simulink model "GWOpss"  (R2025a)
settings: Solver=VariableStepAuto  StartTime=0.0  StopTime=30  RelTol=1e-3
undefined symbols (not defined in the file or in its folder): D1, Delta
libraries: spsExcitationSystemLib x1, spsHydraulicTurbineandGovernorLib x1, spsSynchronousMachinepuStandardLib x1, spsThreePhaseParallelRLCLoadLib x1, spsThreePhaseSeriesRLCBranchLib x1, spsThreePhaseTransformerTwoWindingsLib x1, spsThreePhaseFaultLib x1, spsThreePhaseSourceLib x1, sps_lib x1
settings Model: NumberOfSteps=3  Creator=Amal Ibrahim  LastModifiedBy=Amal Ibrahim
settings DataIOCC: ReturnWorkspaceOutputs=off

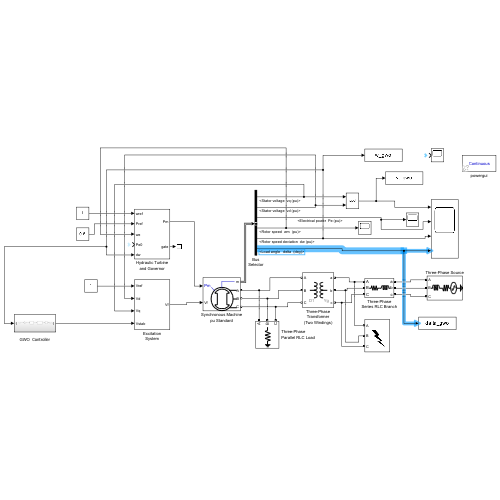
[thumbnail: Simulink's stored preview of the top-level diagram]
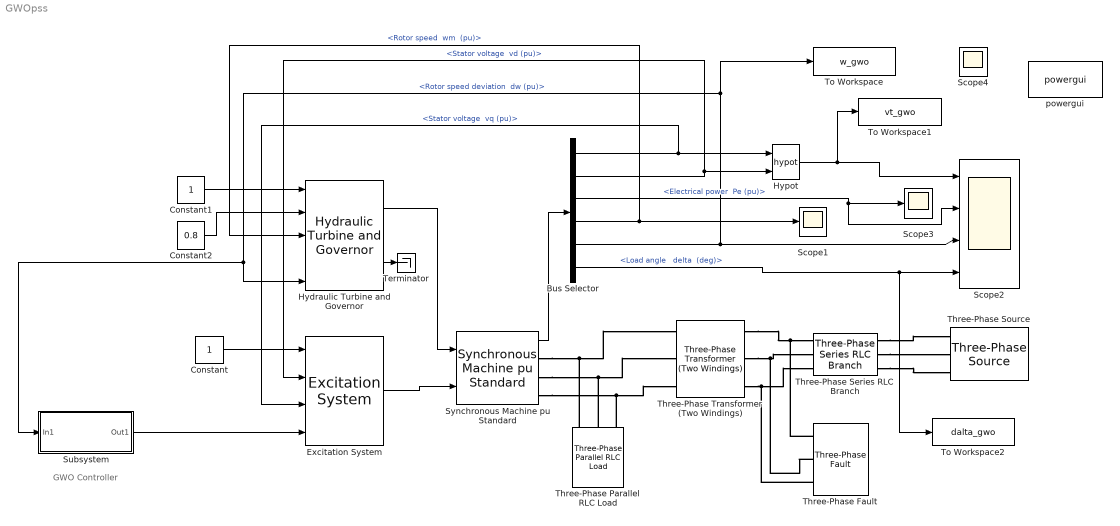
== system GWOpss ==
  note: GWO Controller
  Bus Selector : BusSelector  OutputSignals="dq0 components.Stator voltage  vq (pu),dq0 components.Stator voltage  vd (pu),Mechanical.Electrical power  Pe (pu),Mechanical.Rotor speed  wm  (pu),Mechanical.Rotor speed deviation  dw (pu),Load angle   delta  (deg)"
  Constant : Constant
  Constant1 : Constant
  Constant2 : Constant  Value=0.8
  Excitation System : spsExcitationSystemLib/Excitation System  tr=20e-3  reg=[ 300, 0.001 ]  exc=[ 1, 0 ]  tgr=[ 0, 0 ]  damp=[ 0.01, 0.1 ]  sat=[ 0, 0 ]  lim=[ -11.5, 11.5, 0 ]  v0="[1.0  1.0]"
      settings: LibrarySourceBlock=sps_lib/Electrical Machines/Synchronous Machine Control/Excitation System
  Hydraulic Turbine and Governor : spsHydraulicTurbineandGovernorLib/Hydraulic Turbine and Governor  sm="[ 10/3  0.07 ]"  gate="[  0.01  0.97518  -0.1  0.1 ]"  reg="[  0.05  1.163  0.105  0  0.01  ]"  hyd="[  0  2.67  ]"  dref=0  po=0.8
      settings: LibrarySourceBlock=|
      | sps_lib/Electrical Machines/Synchronous Machine Control/Hydraulic Turbine
      | and Governor
  Hypot : Math  Operator=hypot
  Scope1 : Scope
      settings: ActiveDisplayYMinimum=0.97376212341853119  ActiveDisplayYMaximum=1.0225346527897865
  Scope2 : Scope  NumInputPorts=4
      settings: ActiveDisplayYMinimum=0.13824524933651339  ActiveDisplayYMaximum=1.3474277133856665  DataLoggingVariableName=ScopeData2
  Scope3 : Scope
      settings: ActiveDisplayYMinimum=-1.8399343461680453  ActiveDisplayYMaximum=3.3298477716567159
  Scope4 : Scope
      settings: ActiveDisplayYMinimum=-0.026237876581468769  ActiveDisplayYMaximum=0.022534652789786613  DataLoggingVariableName=ScopeData3
  Subsystem : Subsystem
  Synchronous Machine pu Standard : spsSynchronousMachinepuStandardLib/Synchronous Machine pu Standard  PresetModel=No  MechanicalLoad=Mechanical power Pm  ShowDetailedParameters=on  RotorType=Salient-pole  Units=per unit standard parameters  MeasurementBus=off  NominalParameters=[200E6 13800 60]  Reactances1=[ 1.81, 0.3, 0.23, 1.76, 0.65, 0.25, 0.15 ]  Reactances2=[1.305 0.296 0.252 0.474 0.243 0.18]  dAxisTimeConstants=Short-circuit  qAxisTimeConstants=Open-circuit  TimeConstants1="[ 4.4849  0.0681  0.1  ]"  TimeConstants2=[ 8.0, 0.03, 1.0, 0.07 ]  TimeConstants3="[  4.49  0.0681  0.0513  ]"  TimeConstants4=[ 8.0, 0.03, 0.3371, 0.0295 ]  TimeConstants5=[ 1.01, 0.053, 0.1 ]  TimeConstants6=[ 1.3201, 0.023, 1.0, 0.07 ]  TimeConstants7=[0.012 0.003 0.003]  TimeConstants8=[ 1.3201, 0.0231, 0.3371, 0.0295 ]  StatorResistance=0.037875  Mechanical=[3.2 0 32]  PolePairs=20  InitialConditions="[ 0  0  0  0  0  0  0  0  1 ]"  SetSaturation=off  Saturation=[0.6404,0.7127,0.8441,0.9214,0.9956,1.082,1.19,1.316,1.457;0.7,0.7698,0.8872,0.9466,0.9969,1.046,1.1,1.151,1.201]  LoadFlowParameters=[1,0,0,0,0]  TsPowergui=0  TsBlock=-1  IterativeModel=Trapezoidal non iterative  IterativeDiscreteModel=Trapezoidal non iterative  BusType=PV  Pref=0  Qref=0  Qmin=-inf  Qmax=inf  PLF=0  QLF=0
  Terminator : Terminator
  Three-Phase Parallel RLC Load : spsThreePhaseParallelRLCLoadLib/Three-Phase Parallel RLC Load  LConnTagsString=A|B|C  Configuration=Y (grounded)  NominalVoltage=13.8e3  Vabc=[1e3 1e3 1e3]  Vabcp=[1e3 1e3 1e3]  NominalFrequency=60  UnbalancedPower=off  ActivePower=5e6  InductivePower=0  CapacitivePower=0  Pabc=[10e3 9e3 11e3]  QLabc=[100 90 110]  QCabc=[100 90 110]  Pabcp=[10e3 9e3 11e3]  QLabcp=[100 90 110]  QCabcp=[100 90 110]  Measurements=None  LoadType=constant Z
  Three-Phase Series RLC Branch : spsThreePhaseSeriesRLCBranchLib/Three-Phase Series RLC Branch  LConnTagsString=A|B|C  RConnTagsString=A|B|C  BranchType=RL  Resistance=10  Inductance=0.3  Capacitance=1e-9  Measurements=None
  Three-Phase Transformer (Two Windings) : spsThreePhaseTransformerTwoWindingsLib/Three-Phase Transformer (Two Windings)  Winding1Connection=Delta (D1)  Winding2Connection=Yg  CoreType=Three single-phase transformers  SetSaturation=off  Hysteresis=off  DataFile='hysteresis'  SetInitialFlux=off  Measurements=None  UNITS=pu  NominalPower=[ 210e6 , 60 ]  Winding1=[ 13.8e3 , 0.0027 , 0.08 ]  Winding2=[ 230e3 , 0.0027 , 0.08 ]  Rm=500  Lm=500  L0=0.5  Saturation=[ 0,0 ; 0.0024,1.2 ; 1.0,1.52 ]  InitialFluxes=[ 0.8 , -0.8 , 0.7 ]  BreakLoop=off  DiscreteSolver=Trapezoidal iterative  DataType=off  TransfoNumber=1
  Three-Phase Fault : spsThreePhaseFaultLib/Three-Phase Fault  InitialStates=0  FaultA=on  FaultB=on  FaultC=on  GroundFault=on  SwitchTimes=[10 10.07]  External=off  SwitchStatus=NaN  FaultResistance=0.001  GroundResistance=0.01  SnubberResistance=1e6  SnubberCapacitance=inf  Measurements=None
  Three-Phase Source : spsThreePhaseSourceLib/Three-Phase Source  InternalConnection=Yg  VoltagePhases=off  Voltage=230e3  PhaseAngle=7.3617e-05  Voltage_phases=[25e3 25e3 25e3]/sqrt(3)  PhaseAngles_phases=[0 -120 +120]  Frequency=60  NonIdealSource=on  SpecifyImpedance=off  Resistance=0.8929  Inductance=16.58e-3  ShortCircuitLevel=100e6  BaseVoltage=25e3  XRratio=7  BusType=swing  Pref=10000  Qref=0  Prefabc=[10e3, 10e3, 10e3]  Qrefabc=[0, 0, 0]  Qmin=-Inf  Qmax=Inf
  To Workspace : ToWorkspace  VariableName=w_gwo  SaveFormat=Structure With Time  SampleTime=-1
  To Workspace1 : ToWorkspace  VariableName=vt_gwo  SaveFormat=Structure With Time  SampleTime=-1
  To Workspace2 : ToWorkspace  VariableName=dalta_gwo  SaveFormat=Structure With Time  SampleTime=-1
  powergui : sps_lib/powergui  Priority=1  SimulationMode=Continuous  SampleTime=50e-6  frequency=60  Iterations=50  frequencyindice=60  Pbase=100e6  ErrMax=1e-4  UnitsV=kV  UnitsW=MW  buscounter=0  FunctionMessages=off  echomessages=off  EnableUseOfTLC=off  CurrentSourceSwitches=off  DisableSnubberDevices=off  DisableRonSwitches=off  DisableVfSwitches=off  DisplayEquations=off  AutomaticDiscreteSolvers=off  SolverType=Tustin/Backward Euler (TBE)  Interpol=off  ExternalGateDelay=off  methode=off  Ts=100  x0status=blocks  SPID=on  SwTol=0  HookPort=off  NonlinearTolerance=1e-4  nMaxIteration=100  ContinueOnMaxIteration=off  RestoreLinks=warning  ResistiveCurrentMeasurement=off  Frange=[0:2:500]  Ylog=off  Xlog=on  ShowGrid=off  save=off  variable=ZData  structure=0  ZoomFFT=off  StartTime=0.0  cycles=1  DisplayStyle=1  fundamental=60  FreqAxis=off  MaxFrequency=1000  frequencyindicesteady=1  RmsSteady=1  display=off
  wires:
  Synchronous Machine pu Standard/1 -> Bus Selector/1
  Bus Selector/4 -> Hydraulic Turbine and Governor/3, Scope1/1  "<Rotor speed  wm  (pu)>"
  Bus Selector/1 -> Excitation System/3, Hypot/1  "<Stator voltage  vq (pu)>"
  Bus Selector/2 -> Excitation System/2, Hypot/2  "<Stator voltage  vd (pu)>"
  Bus Selector/3 -> Scope2/2, Scope3/1  "<Electrical power  Pe (pu)>"
  Hydraulic Turbine and Governor/2 -> Terminator/1
  Excitation System/1 -> Synchronous Machine pu Standard/2
  Hydraulic Turbine and Governor/1 -> Synchronous Machine pu Standard/1
  Bus Selector/5 -> To Workspace/1, Subsystem/1(In1), Hydraulic Turbine and Governor/5, Scope2/3  "<Rotor speed deviation  dw (pu)>"
  Constant1/1 -> Hydraulic Turbine and Governor/1
  Constant/1 -> Excitation System/1
  Constant2/1 -> Hydraulic Turbine and Governor/2
  Subsystem/1(Out1) -> Excitation System/4
  Hypot/1 -> To Workspace1/1, Scope2/1
  Bus Selector/6 -> To Workspace2/1, Scope2/4  "<Load angle   delta  (deg)>"
  connections:
  Three-Phase Series RLC Branch/RConn1 -- Three-Phase Source/RConn1
  Three-Phase Series RLC Branch/RConn3 -- Three-Phase Source/RConn3
  Three-Phase Series RLC Branch/RConn2 -- Three-Phase Source/RConn2
  Three-Phase Transformer (Two Windings)/RConn1 -- Three-Phase Fault/LConn1 -- Three-Phase Series RLC Branch/LConn1
  Three-Phase Transformer (Two Windings)/RConn2 -- Three-Phase Fault/LConn2 -- Three-Phase Series RLC Branch/LConn2
  Three-Phase Transformer (Two Windings)/RConn3 -- Three-Phase Fault/LConn3 -- Three-Phase Series RLC Branch/LConn3
  Synchronous Machine pu Standard/RConn1 -- Three-Phase Parallel RLC Load/LConn1 -- Three-Phase Transformer (Two Windings)/LConn1
  Synchronous Machine pu Standard/RConn2 -- Three-Phase Parallel RLC Load/LConn2 -- Three-Phase Transformer (Two Windings)/LConn2
  Synchronous Machine pu Standard/RConn3 -- Three-Phase Parallel RLC Load/LConn3 -- Three-Phase Transformer (Two Windings)/LConn3

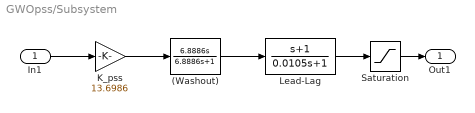
== system GWOpss/Subsystem ==
  In1 : Inport
  "(Washout) " : TransferFcn  Numerator=[6.8886 0]  Denominator=[6.8886 1]
  K_pss : Gain  Gain=13.6986
  Lead-Lag : TransferFcn  Numerator=[1 1]  Denominator=[0.0105 1]
  Saturation : Saturate  UpperLimit=0.1  LowerLimit=-0.1
  Out1 : Outport
  wires:
  K_pss/1 -> "(Washout) "/1
  "(Washout) "/1 -> Lead-Lag/1
  In1/1 -> K_pss/1
  Lead-Lag/1 -> Saturation/1
  Saturation/1 -> Out1/1
